simulink model "Fzgsym_MtrSpd"  (R2022a)
settings: Solver=VariableStepAuto  StartTime=0.0  StopTime=100  RelTol=1e-3
values from neighbouring files (symbols this model uses):
  g = 9.81    [Energiebedarf_single.m]
  m = 1500    [Energiebedarf_single.m]
undefined symbols (not defined in the file or in its folder): air_temp, battPwrChrgLmt, battPwrDischrgLmt, brkprs_front, brkprs_max, brkprs_rear, disk_abore, efficiency, l_CG_rear, mass_veh, mu_kinetic, nmo_rpm, num_mot, num_pads, r_m, trq, trq_eff
libraries: simulink x8, autolibshared x7, autolibmappedmotor x4, autolibutils x1, autolibdatasheetbattery x1
(part 4 of 4)

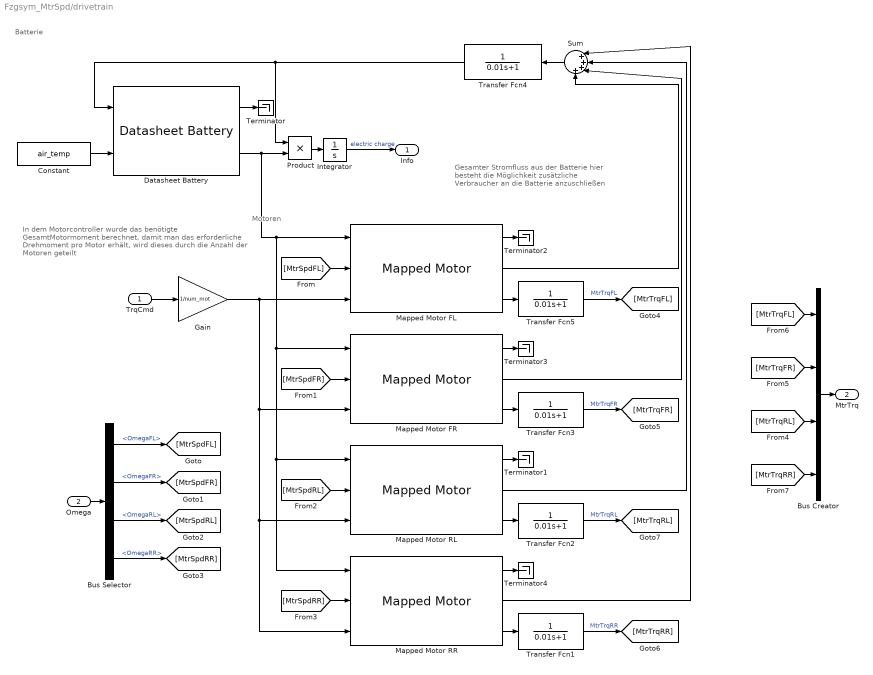
== system Fzgsym_MtrSpd/drivetrain ==
  note: Gesamter Stromfluss aus der Batterie
      | hier besteht die Möglichkeit zusätzliche Verbraucher an die Batterie anzuschließen
  note: Motoren
  note: Batterie
  note: In dem Motorcontroller wurde das benötigte GesamtMotormoment berechnet, damit man das erforderliche Drehmoment pro Motor erhält, wird dieses durch die Anzahl der Motoren geteilt
  TrqCmd : Inport
  Omega : Inport  Port=2
  Bus Creator : BusCreator  Inputs=4
  Bus Selector : BusSelector  OutputSignals=OmegaFL,OmegaFR,OmegaRL,OmegaRR
  Constant : Constant  Value=air_temp
  Datasheet Battery : autolibdatasheetbattery/Datasheet Battery  CapacityCtrl=Parameter  OutputVlt=Unfiltered  BattChargeMax=battchrgmax  Em=[2.8 3.228 3.284 3.361 3.408 3.427 3.472 3.477 3.493 3.504 3.516 3.528 3.537 3.545 3.555 3.561 3.566 3.576 3.587 3.589 3.594 3.6 3.608 3.61 3.616 3.619 3.626 3.632 3.637 3.64 3.645 3.646 3.652 3.655 3.658 3.661 3.664 3.668 3.673 3.678 3.68 3.681 3.686 3.692 3.699 3.702 3.705 3.71 3.717 3.723 3.728 3.733 3.735 3.742 3.749 3.755 3.761 3.768 3.773 3.78 3.791 3.798 3.798 3.814 3.818 3.825 3.841 3.846 3.855 3.863 3.877 3.885 3.894 3.907 3.919 3.926 3.935 3.944 3.954 3.964 3.974 3.988 3.998 4.014 4.029 4.034 4.047 4.065 4.074 4.086 4.097 4.131 4.126 4.138 4.15 4.18 4.174 4.187 4.207 4.231 4.221]  CapLUTBp=[0 0.01 0.02 0.03 0.04 0.05 0.06 0.07 0.08 0.09 0.1 0.11 0.12 0.13 0.14 0.15 0.16 0.17 0.18 0.19 0.2 0.21 0.22 0.23 0.24 0.25 0.26 0.27 0.28 0.29 0.3 0.31 0.32 0.33 0.34 0.35 0.36 0.37 0.38 0.39 0.4 0.41 0.42 0.43 0.44 0.45 0.46 0.47 0.48 0.49 0.5 0.51 0.52 0.53 0.54 0.55 0.56 0.57 0.58 0.59 0.6 0.61 0.62 0.63 0.64 0.65 0.66 0.67 0.68 0.69 0.7 0.71 0.72 0.73 0.74 0.75 0.76 0.77 0.78 0.79 0.8 0.81 0.82 0.83 0.84 0.85 0.86 0.87 0.88 0.89 0.9 0.91 0.92 0.93 0.94 0.95 0.96 0.97 0.98 0.99 1]  RInt=[0.008846 0.009319 0.009027 0.00847 0.01032 0.01314;0.006389 0.006554 0.005553 0.005525 0.006043 0.007805;0.004364 0.004101 0.00406 0.003452 0.003846 0.004517;0.002031 0.002563 0.002532 0.00246 0.002716 0.003047;0.001443 0.001825 0.001795 0.001778 0.001924 0.002234;0.0005603 0.0007192 0.0006887 0.0007557 0.0007355 0.001014;0.001028 0.001338 0.001 0.001536 0.001546 0.002789]  BattTempBp=[243.1 253.1 263.1 273.1 283.1 298.1 313.1]  CapSOCBp=[0 0.2 0.4 0.6 0.8 1]  Ns=num_s  Np=num_p  BattCapInit=100  Tc=1/1000  Vinit=4.221  RefBlkName='autolibdatasheetbattery/Datasheet Battery'
      settings: SourceProductBaseCode=PW
  Gain : Gain  Gain=1/num_mot
  Integrator : Integrator
  Mapped Motor FL : autolibmappedmotor/Mapped Motor  port_config=Speed  param_by=Tabulated torque-speed envelope  w_t=nmo_rad  T_t=trq  torque_max=.1  power_max=30  Tc=Tc  param_loss=Single efficiency measurement  eff=eff_mot  w_eff=nmo_eff  T_eff=T_eff  Piron=P_iron  Pbase=P_base  w_eff_bp=[-800 -400 0 400 800]  T_eff_bp=[0 0.03 0.06 0.09]  Temp_eff_bp=[233.15 293.15 373.15]  losses_table=[1.49 1.67 2.21 3.10; 0.42 0.69 1.14 2.03; 0.06 0.24 0.78 1.68; 0.42 0.69 1.14 2.03; 1.49 1.67 2.21 3.10]  losses_table_3d=cat(3,[1.49 1.67 2.21 3.10; 0.42 0.69 1.14 2.03; 0.06 0.24 0.78 1.68; 0.42 0.69 1.14 2.03; 1.49 1.67 2.21 3.10],[1.49 1.67 2.21 3.10; 0.42 0.69 1.14 2.03; 0.06 0.24 0.78 1.68; 0.42 0.69 1.14 2.03; 1.49 1.67 2.21 3.10],[1.49 1.67 2.21 3.10; 0.42 0.69 1.14 2.03; 0.06 0.24 0.78 1.68; 0.42 0.69 1.14 2.03; 1.49 1.67 2.21 3.10])  efficiency_table=[95 95 95 95; 95 95 95 95; 95 95 95 95; 95 95 95 95; 95 95 95 95]  efficiency_table_3d=cat(3,[95 95 95 95; 95 95 95 95; 95 95 95 95; 95 95 95 95; 95 95 95 95],[95 95 95 95; 95 95 95 95; 95 95 95 95; 95 95 95 95; 95 95 95 95],[95 95 95 95; 95 95 95 95; 95 95 95 95; 95 95 95 95; 95 95 95 95])  J=5e-6  b=1e-5  omega_o=0  T_t_extended=[0 93.3 93.3 93.3 0]  w_t_extended=[-74.895744 -71.261342152 0 71.261342152 74.895744]  KLossIron=0  KLossCopper=0  x_w_eff_vec=[-800 -400 0 400 800]  x_T_eff_vec=[-0.09 -0.06 -0.03 0 0.03 0.06 0.09]  x_tmp_eff_vec=[-0.09 -0.06 -0.03 0 0.03 0.06 0.09]  x_losses_mat=[3.78947368421052 2.52631578947368 1.26315789473684 0 1.2 2.4 3.6;1.89473684210526 1.26315789473684 0.63157894736842 0 0.599999999999999 1.2 1.8;0 0 0 0 0 0 0;1.8 1.2 0.599999999999999 0 0.63157894736842 1.26315789473684 1.89473684210526;3.6 2.4 1.2 0 1.26315789473684 2.52631578947368 3.78947368421052]  x_losses_mat_3d=[37.8947368421052 25.2631578947368 12.6315789473684 0 12 24 36;18.9473684210526 12.6315789473684 6.3157894736842 0 5.99999999999999 12 18;0 0 0 0 0 0 0;18 12 5.99999999999999 0 6.3157894736842 12.6315789473684 18.9473684210526;36 24 12 0 12.6315789473684 25.2631578947368 37.8947368421052]  CalLossMapData={}  CalLossWithTempMapData={}  aMode=1  RefBlkName='autolibmappedmotor/Mapped Motor'
      settings: SourceProductBaseCode=PW,DR,MT,VE
  Mapped Motor FR : autolibmappedmotor/Mapped Motor  port_config=Speed  param_by=Tabulated torque-speed envelope  w_t=nmo_rad  T_t=trq  torque_max=.1  power_max=30  Tc=Tc  param_loss=Single efficiency measurement  eff=eff_mot  w_eff=nmo_eff  T_eff=T_eff  Piron=P_iron  Pbase=P_base  w_eff_bp=[-800 -400 0 400 800]  T_eff_bp=[0 0.03 0.06 0.09]  Temp_eff_bp=[233.15 293.15 373.15]  losses_table=[1.49 1.67 2.21 3.10; 0.42 0.69 1.14 2.03; 0.06 0.24 0.78 1.68; 0.42 0.69 1.14 2.03; 1.49 1.67 2.21 3.10]  losses_table_3d=cat(3,[1.49 1.67 2.21 3.10; 0.42 0.69 1.14 2.03; 0.06 0.24 0.78 1.68; 0.42 0.69 1.14 2.03; 1.49 1.67 2.21 3.10],[1.49 1.67 2.21 3.10; 0.42 0.69 1.14 2.03; 0.06 0.24 0.78 1.68; 0.42 0.69 1.14 2.03; 1.49 1.67 2.21 3.10],[1.49 1.67 2.21 3.10; 0.42 0.69 1.14 2.03; 0.06 0.24 0.78 1.68; 0.42 0.69 1.14 2.03; 1.49 1.67 2.21 3.10])  efficiency_table=[95 95 95 95; 95 95 95 95; 95 95 95 95; 95 95 95 95; 95 95 95 95]  efficiency_table_3d=cat(3,[95 95 95 95; 95 95 95 95; 95 95 95 95; 95 95 95 95; 95 95 95 95],[95 95 95 95; 95 95 95 95; 95 95 95 95; 95 95 95 95; 95 95 95 95],[95 95 95 95; 95 95 95 95; 95 95 95 95; 95 95 95 95; 95 95 95 95])  J=5e-6  b=1e-5  omega_o=0  T_t_extended=[0 93.3 93.3 93.3 0]  w_t_extended=[-74.895744 -71.261342152 0 71.261342152 74.895744]  KLossIron=0  KLossCopper=0  x_w_eff_vec=[-800 -400 0 400 800]  x_T_eff_vec=[-0.09 -0.06 -0.03 0 0.03 0.06 0.09]  x_tmp_eff_vec=[-0.09 -0.06 -0.03 0 0.03 0.06 0.09]  x_losses_mat=[3.78947368421052 2.52631578947368 1.26315789473684 0 1.2 2.4 3.6;1.89473684210526 1.26315789473684 0.63157894736842 0 0.599999999999999 1.2 1.8;0 0 0 0 0 0 0;1.8 1.2 0.599999999999999 0 0.63157894736842 1.26315789473684 1.89473684210526;3.6 2.4 1.2 0 1.26315789473684 2.52631578947368 3.78947368421052]  x_losses_mat_3d=[37.8947368421052 25.2631578947368 12.6315789473684 0 12 24 36;18.9473684210526 12.6315789473684 6.3157894736842 0 5.99999999999999 12 18;0 0 0 0 0 0 0;18 12 5.99999999999999 0 6.3157894736842 12.6315789473684 18.9473684210526;36 24 12 0 12.6315789473684 25.2631578947368 37.8947368421052]  CalLossMapData={}  CalLossWithTempMapData={}  aMode=1  RefBlkName='autolibmappedmotor/Mapped Motor'
      settings: SourceProductBaseCode=PW,DR,MT,VE
  Mapped Motor RL : autolibmappedmotor/Mapped Motor  port_config=Speed  param_by=Tabulated torque-speed envelope  w_t=nmo_rad  T_t=trq  torque_max=.1  power_max=30  Tc=Tc  param_loss=Single efficiency measurement  eff=eff_mot  w_eff=nmo_eff  T_eff=T_eff  Piron=P_iron  Pbase=P_base  w_eff_bp=[-800 -400 0 400 800]  T_eff_bp=[0 0.03 0.06 0.09]  Temp_eff_bp=[233.15 293.15 373.15]  losses_table=[1.49 1.67 2.21 3.10; 0.42 0.69 1.14 2.03; 0.06 0.24 0.78 1.68; 0.42 0.69 1.14 2.03; 1.49 1.67 2.21 3.10]  losses_table_3d=cat(3,[1.49 1.67 2.21 3.10; 0.42 0.69 1.14 2.03; 0.06 0.24 0.78 1.68; 0.42 0.69 1.14 2.03; 1.49 1.67 2.21 3.10],[1.49 1.67 2.21 3.10; 0.42 0.69 1.14 2.03; 0.06 0.24 0.78 1.68; 0.42 0.69 1.14 2.03; 1.49 1.67 2.21 3.10],[1.49 1.67 2.21 3.10; 0.42 0.69 1.14 2.03; 0.06 0.24 0.78 1.68; 0.42 0.69 1.14 2.03; 1.49 1.67 2.21 3.10])  efficiency_table=[95 95 95 95; 95 95 95 95; 95 95 95 95; 95 95 95 95; 95 95 95 95]  efficiency_table_3d=cat(3,[95 95 95 95; 95 95 95 95; 95 95 95 95; 95 95 95 95; 95 95 95 95],[95 95 95 95; 95 95 95 95; 95 95 95 95; 95 95 95 95; 95 95 95 95],[95 95 95 95; 95 95 95 95; 95 95 95 95; 95 95 95 95; 95 95 95 95])  J=5e-6  b=1e-5  omega_o=0  T_t_extended=[0 93.3 93.3 93.3 0]  w_t_extended=[-74.895744 -71.261342152 0 71.261342152 74.895744]  KLossIron=0  KLossCopper=0  x_w_eff_vec=[-800 -400 0 400 800]  x_T_eff_vec=[-0.09 -0.06 -0.03 0 0.03 0.06 0.09]  x_tmp_eff_vec=[-0.09 -0.06 -0.03 0 0.03 0.06 0.09]  x_losses_mat=[3.78947368421052 2.52631578947368 1.26315789473684 0 1.2 2.4 3.6;1.89473684210526 1.26315789473684 0.63157894736842 0 0.599999999999999 1.2 1.8;0 0 0 0 0 0 0;1.8 1.2 0.599999999999999 0 0.63157894736842 1.26315789473684 1.89473684210526;3.6 2.4 1.2 0 1.26315789473684 2.52631578947368 3.78947368421052]  x_losses_mat_3d=[37.8947368421052 25.2631578947368 12.6315789473684 0 12 24 36;18.9473684210526 12.6315789473684 6.3157894736842 0 5.99999999999999 12 18;0 0 0 0 0 0 0;18 12 5.99999999999999 0 6.3157894736842 12.6315789473684 18.9473684210526;36 24 12 0 12.6315789473684 25.2631578947368 37.8947368421052]  CalLossMapData={}  CalLossWithTempMapData={}  aMode=1  RefBlkName='autolibmappedmotor/Mapped Motor'
      settings: SourceProductBaseCode=PW,DR,MT,VE
  Mapped Motor RR : autolibmappedmotor/Mapped Motor  port_config=Speed  param_by=Tabulated torque-speed envelope  w_t=nmo_rad  T_t=trq  torque_max=.1  power_max=30  Tc=Tc  param_loss=Single efficiency measurement  eff=eff_mot  w_eff=nmo_eff  T_eff=T_eff  Piron=P_iron  Pbase=P_base  w_eff_bp=[-800 -400 0 400 800]  T_eff_bp=[0 0.03 0.06 0.09]  Temp_eff_bp=[233.15 293.15 373.15]  losses_table=[1.49 1.67 2.21 3.10; 0.42 0.69 1.14 2.03; 0.06 0.24 0.78 1.68; 0.42 0.69 1.14 2.03; 1.49 1.67 2.21 3.10]  losses_table_3d=cat(3,[1.49 1.67 2.21 3.10; 0.42 0.69 1.14 2.03; 0.06 0.24 0.78 1.68; 0.42 0.69 1.14 2.03; 1.49 1.67 2.21 3.10],[1.49 1.67 2.21 3.10; 0.42 0.69 1.14 2.03; 0.06 0.24 0.78 1.68; 0.42 0.69 1.14 2.03; 1.49 1.67 2.21 3.10],[1.49 1.67 2.21 3.10; 0.42 0.69 1.14 2.03; 0.06 0.24 0.78 1.68; 0.42 0.69 1.14 2.03; 1.49 1.67 2.21 3.10])  efficiency_table=[95 95 95 95; 95 95 95 95; 95 95 95 95; 95 95 95 95; 95 95 95 95]  efficiency_table_3d=cat(3,[95 95 95 95; 95 95 95 95; 95 95 95 95; 95 95 95 95; 95 95 95 95],[95 95 95 95; 95 95 95 95; 95 95 95 95; 95 95 95 95; 95 95 95 95],[95 95 95 95; 95 95 95 95; 95 95 95 95; 95 95 95 95; 95 95 95 95])  J=5e-6  b=1e-5  omega_o=0  T_t_extended=[0 93.3 93.3 93.3 0]  w_t_extended=[-74.895744 -71.261342152 0 71.261342152 74.895744]  KLossIron=0  KLossCopper=0  x_w_eff_vec=[-800 -400 0 400 800]  x_T_eff_vec=[-0.09 -0.06 -0.03 0 0.03 0.06 0.09]  x_tmp_eff_vec=[-0.09 -0.06 -0.03 0 0.03 0.06 0.09]  x_losses_mat=[3.78947368421052 2.52631578947368 1.26315789473684 0 1.2 2.4 3.6;1.89473684210526 1.26315789473684 0.63157894736842 0 0.599999999999999 1.2 1.8;0 0 0 0 0 0 0;1.8 1.2 0.599999999999999 0 0.63157894736842 1.26315789473684 1.89473684210526;3.6 2.4 1.2 0 1.26315789473684 2.52631578947368 3.78947368421052]  x_losses_mat_3d=[37.8947368421052 25.2631578947368 12.6315789473684 0 12 24 36;18.9473684210526 12.6315789473684 6.3157894736842 0 5.99999999999999 12 18;0 0 0 0 0 0 0;18 12 5.99999999999999 0 6.3157894736842 12.6315789473684 18.9473684210526;36 24 12 0 12.6315789473684 25.2631578947368 37.8947368421052]  CalLossMapData={}  CalLossWithTempMapData={}  aMode=1  RefBlkName='autolibmappedmotor/Mapped Motor'
      settings: SourceProductBaseCode=PW,DR,MT,VE
  Product : Product
  Sum : Sum  Inputs=|++++
  Terminator{,1..4} (5 alike) : Terminator
  Transfer Fcn{1..5} (5 alike) : TransferFcn  Denominator=[0.01 1]
  Info : Outport
  MtrTrq : Outport  Port=2
  wires:
  Mapped Motor RR/1 -> Terminator4/1
  [MtrSpdRL] -> Mapped Motor RL/2
  Sum/1 -> Transfer Fcn4/1
  Constant/1 -> Datasheet Battery/2
  [MtrSpdFL] -> Mapped Motor FL/2
  Mapped Motor RL/3 -> Transfer Fcn2/1
  Mapped Motor RR/3 -> Transfer Fcn1/1
  Mapped Motor FR/3 -> Transfer Fcn3/1
  [MtrSpdFR] -> Mapped Motor FR/2
  [MtrSpdRR] -> Mapped Motor RR/2
  Mapped Motor FR/1 -> Terminator3/1
  Mapped Motor FL/1 -> Terminator2/1
  Mapped Motor RL/1 -> Terminator1/1
  Mapped Motor FL/3 -> Transfer Fcn5/1
  Datasheet Battery/1 -> Terminator/1
  Transfer Fcn4/1 -> Product/1, Datasheet Battery/1
  Mapped Motor FL/2 -> Sum/4
  Mapped Motor FR/2 -> Sum/3
  Mapped Motor RL/2 -> Sum/2
  Mapped Motor RR/2 -> Sum/1
  TrqCmd/1 -> Gain/1
  Gain/1 -> Mapped Motor RR/3, Mapped Motor RL/3, Mapped Motor FR/3, Mapped Motor FL/3
  Transfer Fcn5/1 -> [MtrTrqFL]  "MtrTrqFL"
  Transfer Fcn3/1 -> [MtrTrqFR]  "MtrTrqFR"
  Transfer Fcn2/1 -> [MtrTrqRL]  "MtrTrqRL"
  Transfer Fcn1/1 -> [MtrTrqRR]  "MtrTrqRR"
  Datasheet Battery/2 -> Product/2, Mapped Motor FL/1, Mapped Motor FR/1, Mapped Motor RR/1, Mapped Motor RL/1
  Omega/1 -> Bus Selector/1
  Bus Selector/1 -> [MtrSpdFL]  "<OmegaFL>"
  Bus Selector/4 -> [MtrSpdRR]  "<OmegaRR>"
  Bus Selector/2 -> [MtrSpdFR]  "<OmegaFR>"
  Bus Selector/3 -> [MtrSpdRL]  "<OmegaRL>"
  Product/1 -> Integrator/1
  Integrator/1 -> Info/1  "electric charge"
  Bus Creator/1 -> MtrTrq/1
  [MtrTrqRR] -> Bus Creator/4
  [MtrTrqRL] -> Bus Creator/3
  [MtrTrqFR] -> Bus Creator/2
  [MtrTrqFL] -> Bus Creator/1

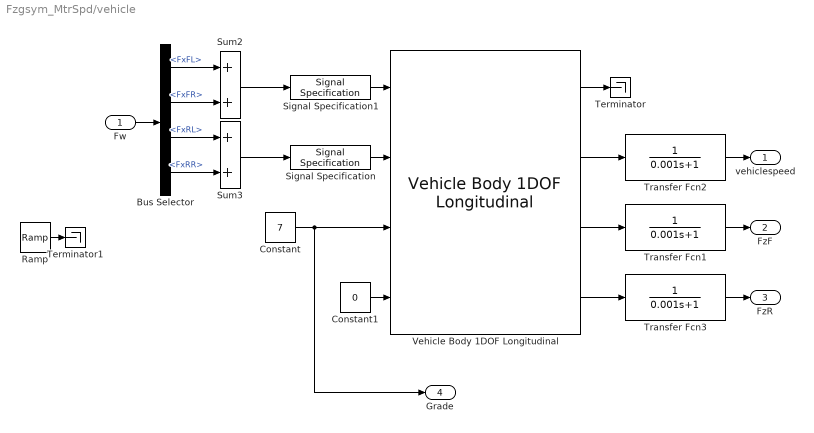
== system Fzgsym_MtrSpd/vehicle ==
  Fw : Inport
  Bus Selector : BusSelector  OutputSignals=FxFL,FxFR,FxRL,FxRR
  Constant : Constant  Value=7
  Constant1 : Constant  Value=0
  Ramp : simulink/Sources/Ramp  slope=0.1  start=0  InitialOutput=0
  Signal Specification : SignalSpecification  Unit=N
  Signal Specification1 : SignalSpecification  Unit=N
  Sum2 : Sum
  Sum3 : Sum
  Terminator : Terminator
  Terminator1 : Terminator
  Transfer Fcn1 : TransferFcn  Denominator=[0.001 1]
  Transfer Fcn2 : TransferFcn  Denominator=[0.001 1]
  Transfer Fcn3 : TransferFcn  Denominator=[0.001 1]
  Vehicle Body 1DOF Longitudinal : autolibshared/Vehicle Body 1DOF Longitudinal  VariantControl=SL  extFMode=off  extMMode=off  extTamb=off  wind3D=off  aMode=1  NF=2  NR=2  m=mass_veh  a=l_CG_front  b=l_CG_rear  h=h_CG  Cd=c_d  Cl=c_l  Cpm=c_pm  Af=A_f  x_o=x_o  xdot_o=xdot_o  Pabs=abs_pressure  T=air_temp  g=g
      settings: SourceProductBaseCode=PW,DR,MT,VE
  vehiclespeed : Outport
  FzF : Outport  Port=2
  FzR : Outport  Port=3
  Grade : Outport  Port=4
  wires:
  Signal Specification1/1 -> Vehicle Body 1DOF Longitudinal/1
  Bus Selector/4 -> Sum3/2  "<FxRR>"
  Sum3/1 -> Signal Specification/1
  Constant1/1 -> Vehicle Body 1DOF Longitudinal/4
  Signal Specification/1 -> Vehicle Body 1DOF Longitudinal/2
  Sum2/1 -> Signal Specification1/1
  Vehicle Body 1DOF Longitudinal/4 -> Transfer Fcn3/1
  Vehicle Body 1DOF Longitudinal/2 -> Transfer Fcn2/1
  Vehicle Body 1DOF Longitudinal/3 -> Transfer Fcn1/1
  Vehicle Body 1DOF Longitudinal/1 -> Terminator/1
  Transfer Fcn2/1 -> vehiclespeed/1
  Transfer Fcn1/1 -> FzF/1
  Transfer Fcn3/1 -> FzR/1
  Fw/1 -> Bus Selector/1
  Bus Selector/1 -> Sum2/1  "<FxFL>"
  Bus Selector/2 -> Sum2/2  "<FxFR>"
  Bus Selector/3 -> Sum3/1  "<FxRL>"
  Ramp/1 -> Terminator1/1
  Constant/1 -> Vehicle Body 1DOF Longitudinal/3, Grade/1

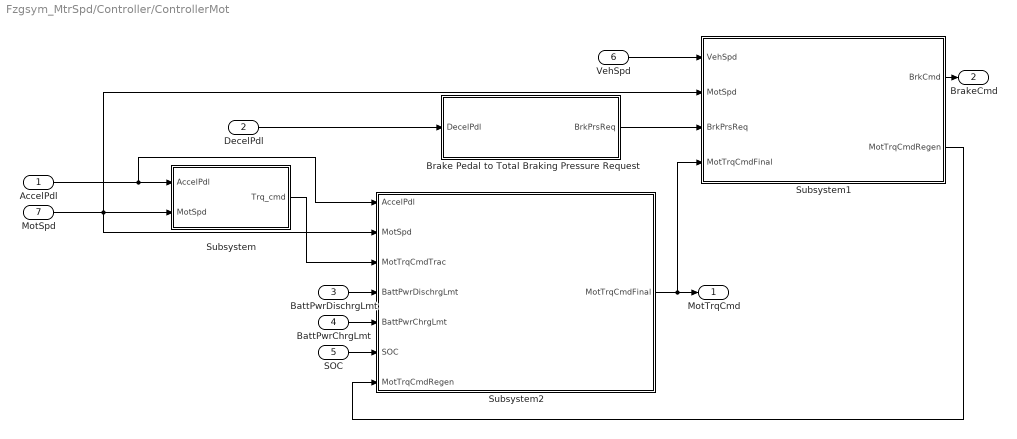
== system Fzgsym_MtrSpd/Controller/ControllerMot ==
  AccelPdl : Inport
  DecelPdl : Inport  Port=2
  BattPwrDischrgLmt : Inport  Port=3
  BattPwrChrgLmt : Inport  Port=4
  SOC : Inport  Port=5
  VehSpd : Inport  Port=6
  MotSpd : Inport  Port=7
  Brake Pedal to Total Braking Pressure Request : Subsystem
  Subsystem : Subsystem
  Subsystem1 : Subsystem
  Subsystem2 : Subsystem
  MotTrqCmd : Outport
  BrakeCmd : Outport  Port=2
  wires:
  Subsystem1/1(BrkCmd) -> BrakeCmd/1
  Subsystem1/2(MotTrqCmdRegen) -> Subsystem2/7(MotTrqCmdRegen)
  BattPwrChrgLmt/1 -> Subsystem2/5(BattPwrChrgLmt)
  VehSpd/1 -> Subsystem1/1(VehSpd)
  MotSpd/1 -> Subsystem2/2(MotSpd), Subsystem/2(MotSpd), Subsystem1/2(MotSpd)
  SOC/1 -> Subsystem2/6(SOC)
  AccelPdl/1 -> Subsystem2/1(AccelPdl), Subsystem/1(AccelPdl)
  BattPwrDischrgLmt/1 -> Subsystem2/4(BattPwrDischrgLmt)
  Subsystem/1(Trq_cmd) -> Subsystem2/3(MotTrqCmdTrac)
  Subsystem2/1(MotTrqCmdFinal) -> Subsystem1/4(MotTrqCmdFinal), MotTrqCmd/1
  Brake Pedal to Total Braking Pressure Request/1(BrkPrsReq) -> Subsystem1/3(BrkPrsReq)
  DecelPdl/1 -> Brake Pedal to Total Braking Pressure Request/1(DecelPdl)

== system Fzgsym_MtrSpd/Controller/ControllerMot/Brake Pedal to Total Braking Pressure Request ==
  note: Bremspedalstellung wird mit dem maximal möglichen Bremsdruck multipliziert, um den benötigten Bremsdruck zu berechnen
  DecelPdl : Inport
  Constant5 : Constant  Value=brkprs_max
  Product1 : Product
  BrkPrsReq : Outport
  wires:
  Constant5/1 -> Product1/2
  Product1/1 -> BrkPrsReq/1
  DecelPdl/1 -> Product1/1

== system Fzgsym_MtrSpd/Controller/ControllerMot/Subsystem ==
  note: (Hinweis: hier wird das Motormoment aller Motoren addiert um somit das Gesamtmotormoment zu berechnen)
  note: Gaspedalstellung wird mit dem zum aktuellen Zeitpunkt maximal möglichen Motormoment multipliziert, um daraus das benötigte Motormoment zu berechnen
  AccelPdl : Inport
  MotSpd : Inport  Port=2
  Drehmoment über Drehzahl : Lookup_n-D  NumberOfTableDimensions=1  BreakpointsForDimension1=nmo_rpm  BreakpointsForDimension3=[5, 7]  Table=trq*num_mot  InternalRulePriority=Speed  RndMeth=Simplest
  Product : Product
  rads_to_rpm : Gain  Gain=30/pi
  Trq_cmd : Outport
  wires:
  Product/1 -> Trq_cmd/1  "Trq_cmd"
  AccelPdl/1 -> Product/1
  rads_to_rpm/1 -> Drehmoment über Drehzahl/1
  Drehmoment über Drehzahl/1 -> Product/2
  MotSpd/1 -> rads_to_rpm/1

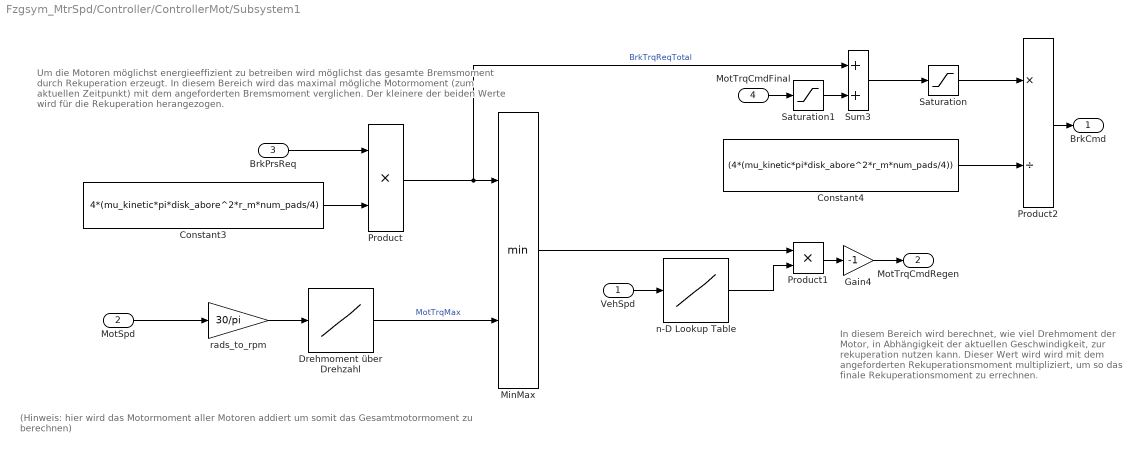
== system Fzgsym_MtrSpd/Controller/ControllerMot/Subsystem1 ==
  note: In diesem Bereich wird berechnet, wie viel Drehmoment der Motor, in Abhängigkeit der aktuellen Geschwindigkeit, zur rekuperation nutzen kann. Dieser Wert wird wird mit dem angeforderten Rekuperationsmoment multipliziert, um so das finale Rekuperationsmoment zu errechnen.
  note: Um die Motoren möglichst energieeffizient zu betreiben wird möglichst das gesamte Bremsmoment durch Rekuperation erzeugt.
      | In diesem Bereich wird das maximal mögliche Motormoment (zum aktuellen Zeitpunkt) mit dem angeforderten Bremsmoment verglichen. Der kleinere der beiden Werte wird für die Rekuperation herangezogen.
  note: (Hinweis: hier wird das Motormoment aller Motoren addiert um somit das Gesamtmotormoment zu berechnen)
  VehSpd : Inport
  MotSpd : Inport  Port=2
  BrkPrsReq : Inport  Port=3
  MotTrqCmdFinal : Inport  Port=4
  Constant3 : Constant  Value=4*(mu_kinetic*pi*disk_abore^2*r_m*num_pads/4)
  Constant4 : Constant  Value=(4*(mu_kinetic*pi*disk_abore^2*r_m*num_pads/4))
  Drehmoment über Drehzahl : Lookup_n-D  NumberOfTableDimensions=1  BreakpointsForDimension1=nmo_rpm  BreakpointsForDimension3=[5, 7]  Table=trq*num_mot  InternalRulePriority=Speed  RndMeth=Simplest
  Gain4 : Gain  Gain=-1
  MinMax : MinMax  Inputs=2
  Product : Product
  Product1 : Product
  Product2 : Product  Inputs=*/
  Saturation : Saturate  UpperLimit=inf  LowerLimit=0
  Saturation1 : Saturate  UpperLimit=0  LowerLimit=-inf
  Sum3 : Sum
  n-D Lookup Table : Lookup_n-D  NumberOfTableDimensions=1  BreakpointsForDimension1=[5 9]  BreakpointsForDimension3=[5, 7]  Table=[0 1]  ExtrapMethod=Clip  UseLastTableValue=on  InternalRulePriority=Speed  RndMeth=Simplest
  rads_to_rpm : Gain  Gain=30/pi
  BrkCmd : Outport
  MotTrqCmdRegen : Outport  Port=2
  wires:
  Sum3/1 -> Saturation/1
  MinMax/1 -> Product1/1
  BrkPrsReq/1 -> Product/1
  Constant4/1 -> Product2/2
  Product1/1 -> Gain4/1
  MotSpd/1 -> rads_to_rpm/1
  Drehmoment über Drehzahl/1 -> MinMax/2  "MotTrqMax"
  Product/1 -> Sum3/1, MinMax/1  "BrkTrqReqTotal"
  Saturation/1 -> Product2/1
  Constant3/1 -> Product/2
  rads_to_rpm/1 -> Drehmoment über Drehzahl/1
  VehSpd/1 -> n-D Lookup Table/1
  Gain4/1 -> MotTrqCmdRegen/1
  MotTrqCmdFinal/1 -> Saturation1/1
  Product2/1 -> BrkCmd/1
  Saturation1/1 -> Sum3/2
  n-D Lookup Table/1 -> Product1/2

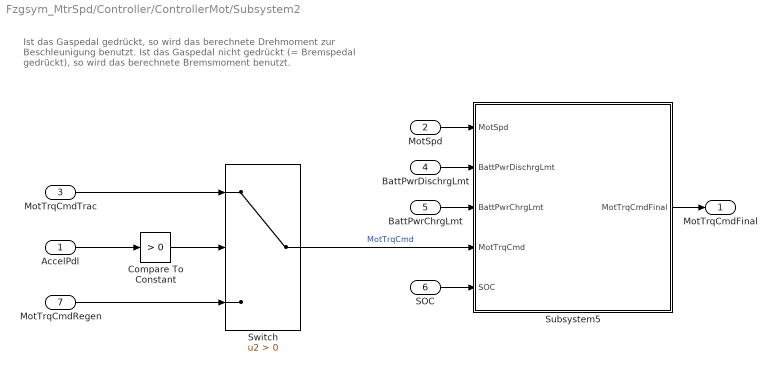
== system Fzgsym_MtrSpd/Controller/ControllerMot/Subsystem2 ==
  note: Ist das Gaspedal gedrückt, so wird das berechnete Drehmoment zur Beschleunigung benutzt. Ist das Gaspedal nicht gedrückt (= Bremspedal gedrückt), so wird das berechnete Bremsmoment benutzt.
  AccelPdl : Inport
  MotSpd : Inport  Port=2
  MotTrqCmdTrac : Inport  Port=3
  BattPwrDischrgLmt : Inport  Port=4
  BattPwrChrgLmt : Inport  Port=5
  SOC : Inport  Port=6
  MotTrqCmdRegen : Inport  Port=7
  Compare To Constant : simulink/Logic and Bit Operations/Compare To Constant  relop=>  const=0  OutDataTypeStr=boolean
  Subsystem5 : Subsystem
  Switch : Switch  Criteria=u2 > Threshold  SaturateOnIntegerOverflow=off  InputSameDT=off
  MotTrqCmdFinal : Outport
  wires:
  Subsystem5/1(MotTrqCmdFinal) -> MotTrqCmdFinal/1
  SOC/1 -> Subsystem5/5(SOC)
  Switch/1 -> Subsystem5/4(MotTrqCmd)  "MotTrqCmd"
  Compare To Constant/1 -> Switch/2
  BattPwrDischrgLmt/1 -> Subsystem5/2(BattPwrDischrgLmt)
  AccelPdl/1 -> Compare To Constant/1
  BattPwrChrgLmt/1 -> Subsystem5/3(BattPwrChrgLmt)
  MotSpd/1 -> Subsystem5/1(MotSpd)
  MotTrqCmdRegen/1 -> Switch/3
  MotTrqCmdTrac/1 -> Switch/1

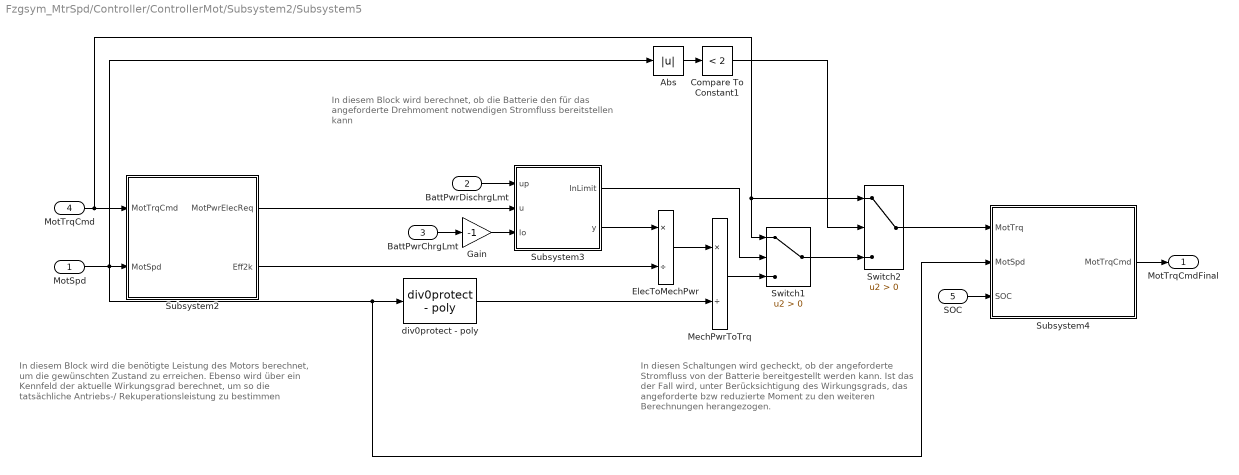
== system Fzgsym_MtrSpd/Controller/ControllerMot/Subsystem2/Subsystem5 ==
  note: In diesem Block wird die benötigte Leistung des Motors berechnet, um die gewünschten Zustand zu erreichen. Ebenso wird über ein Kennfeld der aktuelle Wirkungsgrad berechnet, um so die tatsächliche Antriebs-/ Rekuperationsleistung zu bestimmen
  note: In diesen Schaltungen wird gecheckt, ob der angeforderte Stromfluss von der Batterie bereitgestellt werden kann. Ist das der Fall wird, unter Berücksichtigung des Wirkungsgrads, das angeforderte bzw reduzierte Moment zu den weiteren Berechnungen herangezogen.
  note: In diesem Block wird berechnet, ob die Batterie den für das angeforderte Drehmoment notwendigen Stromfluss bereitstellen kann
  MotSpd : Inport
  BattPwrDischrgLmt : Inport  Port=2
  BattPwrChrgLmt : Inport  Port=3
  MotTrqCmd : Inport  Port=4
  SOC : Inport  Port=5
  Abs : Abs  SaturateOnIntegerOverflow=off
  Compare To Constant1 : simulink/Logic and Bit Operations/Compare To Constant  relop=<  const=2  OutDataTypeStr=boolean
  ElecToMechPwr : Product  Inputs=*/
  Gain : Gain  Gain=-1
  MechPwrToTrq : Product  Inputs=*/
  Subsystem2 : Subsystem
  Subsystem3 : Subsystem
  Subsystem4 : Subsystem
  Switch1 : Switch  Criteria=u2 > Threshold  SaturateOnIntegerOverflow=off  InputSameDT=off
  Switch2 : Switch  Criteria=u2 > Threshold  SaturateOnIntegerOverflow=off  InputSameDT=off
  div0protect - poly : autolibutils/div0protect - poly  thresh=2  ZeroCross1=off  aMode=aMode
      settings: SourceProductBaseCode=PW,DR,MT,VE
  MotTrqCmdFinal : Outport
  wires:
  Subsystem2/1(MotPwrElecReq) -> Subsystem3/2(u)
  MotSpd/1 -> Subsystem4/2(MotSpd), div0protect - poly/1, Abs/1, Subsystem2/2(MotSpd)
  BattPwrDischrgLmt/1 -> Subsystem3/1(up)
  MotTrqCmd/1 -> Switch1/1, Switch2/1, Subsystem2/1(MotTrqCmd)
  div0protect - poly/1 -> MechPwrToTrq/2
  MechPwrToTrq/1 -> Switch1/3
  Switch2/1 -> Subsystem4/1(MotTrq)
  Subsystem2/2(Eff2k) -> ElecToMechPwr/2
  Subsystem3/1(InLimit) -> Switch1/2
  ElecToMechPwr/1 -> MechPwrToTrq/1
  Compare To Constant1/1 -> Switch2/2
  SOC/1 -> Subsystem4/3(SOC)
  Abs/1 -> Compare To Constant1/1
  Switch1/1 -> Switch2/3
  Subsystem3/2(y) -> ElecToMechPwr/1
  BattPwrChrgLmt/1 -> Gain/1
  Subsystem4/1(MotTrqCmd) -> MotTrqCmdFinal/1
  Gain/1 -> Subsystem3/3(lo)

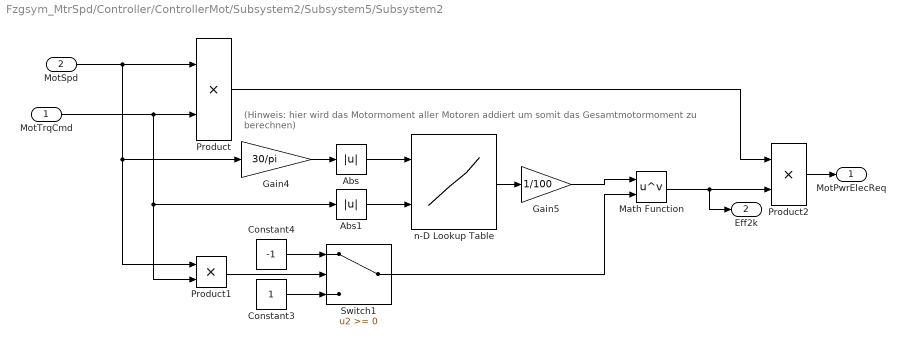
== system Fzgsym_MtrSpd/Controller/ControllerMot/Subsystem2/Subsystem5/Subsystem2 ==
  note: (Hinweis: hier wird das Motormoment aller Motoren addiert um somit das Gesamtmotormoment zu berechnen)
  MotTrqCmd : Inport
  MotSpd : Inport  Port=2
  Abs : Abs  SaturateOnIntegerOverflow=off
  Abs1 : Abs  SaturateOnIntegerOverflow=off
  Constant3 : Constant
  Constant4 : Constant  Value=-1
  Gain4 : Gain  Gain=30/pi
  Gain5 : Gain  Gain=1/100
  Math Function : Math  Operator=pow  SignedPower=on  OutputSignalType=real
  Product : Product
  Product1 : Product
  Product2 : Product
  Switch1 : Switch  SaturateOnIntegerOverflow=off  InputSameDT=off
  n-D Lookup Table : Lookup_n-D  BreakpointsForDimension1=nmo_rpm  BreakpointsForDimension2=trq_eff  BreakpointsForDimension3=[5, 7]  Table=efficiency  InternalRulePriority=Speed  RndMeth=Simplest
      settings: InputPortMap=u0,u1
  MotPwrElecReq : Outport
  Eff2k : Outport  Port=2
  wires:
  Constant4/1 -> Switch1/1
  Switch1/1 -> Math Function/2
  Product1/1 -> Switch1/2
  Constant3/1 -> Switch1/3
  Gain5/1 -> Math Function/1
  Product/1 -> Product2/1
  Abs1/1 -> n-D Lookup Table/2
  MotTrqCmd/1 -> Abs1/1, Product1/2, Product/2
  MotSpd/1 -> Product/1, Product1/1, Gain4/1
  Abs/1 -> n-D Lookup Table/1
  n-D Lookup Table/1 -> Gain5/1
  Gain4/1 -> Abs/1
  Math Function/1 -> Eff2k/1, Product2/2
  Product2/1 -> MotPwrElecReq/1

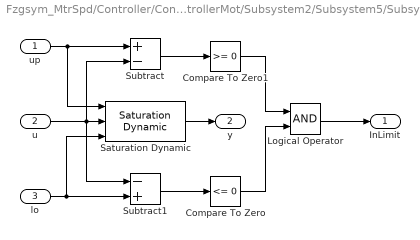
== system Fzgsym_MtrSpd/Controller/ControllerMot/Subsystem2/Subsystem5/Subsystem3 ==
  up : Inport
  u : Inport  Port=2
  lo : Inport  Port=3
  Compare To Zero : simulink/Logic and Bit Operations/Compare To Zero  relop=<=  OutDataTypeStr=boolean
  Compare To Zero1 : simulink/Logic and Bit Operations/Compare To Zero  relop=>=  OutDataTypeStr=boolean
  Logical Operator : Logic  AllPortsSameDT=off  OutDataTypeStr=boolean
  Saturation Dynamic : simulink/Discontinuities/Saturation Dynamic  OutMin=[]  OutMax=[]  OutDataTypeStr=Inherit: Same as second input  OutDataType=fixdt(1, 16)  OutScaling=2^-10  DoSatur=off
  Subtract : Sum  Inputs=+-
  Subtract1 : Sum  Inputs=-+
  InLimit : Outport
  y : Outport  Port=2
  wires:
  Subtract1/1 -> Compare To Zero/1
  Logical Operator/1 -> InLimit/1
  Subtract/1 -> Compare To Zero1/1
  Compare To Zero1/1 -> Logical Operator/1
  Compare To Zero/1 -> Logical Operator/2
  lo/1 -> Saturation Dynamic/3, Subtract1/2
  up/1 -> Saturation Dynamic/1, Subtract/1
  u/1 -> Subtract1/1, Subtract/2, Saturation Dynamic/2
  Saturation Dynamic/1 -> y/1

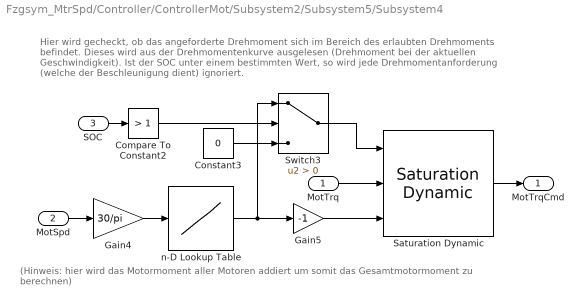
== system Fzgsym_MtrSpd/Controller/ControllerMot/Subsystem2/Subsystem5/Subsystem4 ==
  note: Hier wird gecheckt, ob das angeforderte Drehmoment sich im Bereich des erlaubten Drehmoments befindet. Dieses wird aus der Drehmomentenkurve ausgelesen (Drehmoment bei der aktuellen Geschwindigkeit).
      | Ist der SOC unter einem bestimmten Wert, so wird jede Drehmomentanforderung (welche der Beschleunigung dient) ignoriert.
  note: (Hinweis: hier wird das Motormoment aller Motoren addiert um somit das Gesamtmotormoment zu berechnen)
  MotTrq : Inport
  MotSpd : Inport  Port=2
  SOC : Inport  Port=3
  Compare To Constant2 : simulink/Logic and Bit Operations/Compare To Constant  relop=>  const=1  OutDataTypeStr=boolean
  Constant3 : Constant  Value=0
  Gain4 : Gain  Gain=30/pi
  Gain5 : Gain  Gain=-1
  Saturation Dynamic : simulink/Discontinuities/Saturation Dynamic  OutMin=[]  OutMax=[]  OutDataTypeStr=Inherit: Same as second input  OutDataType=fixdt(1, 16)  OutScaling=2^-10  DoSatur=off
  Switch3 : Switch  Criteria=u2 > Threshold  SaturateOnIntegerOverflow=off  InputSameDT=off
  n-D Lookup Table : Lookup_n-D  NumberOfTableDimensions=1  BreakpointsForDimension1=nmo_rpm  BreakpointsForDimension3=[5, 7]  Table=trq*num_mot  InternalRulePriority=Speed  RndMeth=Simplest
  MotTrqCmd : Outport
  wires:
  n-D Lookup Table/1 -> Gain5/1, Switch3/1
  Constant3/1 -> Switch3/3
  MotSpd/1 -> Gain4/1
  Switch3/1 -> Saturation Dynamic/1
  Compare To Constant2/1 -> Switch3/2
  Gain4/1 -> n-D Lookup Table/1
  Gain5/1 -> Saturation Dynamic/3
  SOC/1 -> Compare To Constant2/1
  Saturation Dynamic/1 -> MotTrqCmd/1
  MotTrq/1 -> Saturation Dynamic/2
